simulink model "pruebaudpreceive"  (R2025a)
settings: Solver=FixedStepAuto  StartTime=0.0  StopTime=inf  FixedStep=0.001  RelTol=1e-3
libraries: etargetslib x1, dspnetwork x1
settings Model: Creator=aero  LastModifiedBy=aero

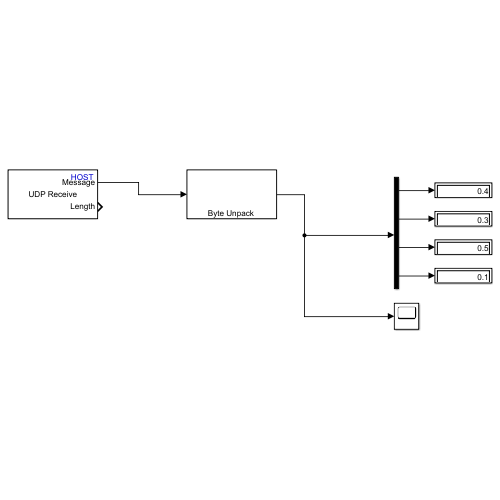
[thumbnail: Simulink's stored preview of the top-level diagram]
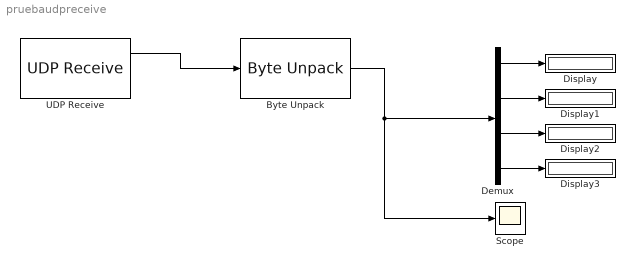
== system pruebaudpreceive ==
  Byte Unpack : etargetslib/Byte Unpack  dimensions={[4]}  datatypes={'double'}  byteAlign=8
      settings: LibrarySourceBlock=embeddedtargetslib/Host Communication/Byte Unpack
  Demux : Demux
  Display{,1..3} (4 alike) : Display
  Scope : Scope
      settings: ActiveDisplayYMinimum=-1.2499999148694405  ActiveDisplayYMaximum=1.2499999903536541
  UDP Receive : dspnetwork/UDP Receive  localURL='0.0.0.0'  localPort=25000  remoteURL='0.0.0.0'  remotePort=-1  recvBufferSize=8192  dims=32  signalDatatype=uint8  isComplex=off  isVarSize=off  showBlockingTime=on  blockingTime=0  sampletime=0.001  blockPlatform=HOST
      settings: LibrarySourceBlock=embeddedtargetslib/Host Communication/UDP Receive
  wires:
  UDP Receive/1 -> Byte Unpack/1
  Byte Unpack/1 -> Demux/1, Scope/1
  Demux/1 -> Display/1
  Demux/2 -> Display1/1
  Demux/3 -> Display2/1
  Demux/4 -> Display3/1
